simulink model "qpsk"  (Simulink 6.0)
settings: Solver=ode45  StartTime=0.0  StopTime=10.0  RelTol=1e-3
libraries: commsink2 x3, commdigbbndpm2 x2, commchan2 x1, commfilt2 x1, commrandsrc2 x1
settings Model: LastModifiedBy=student

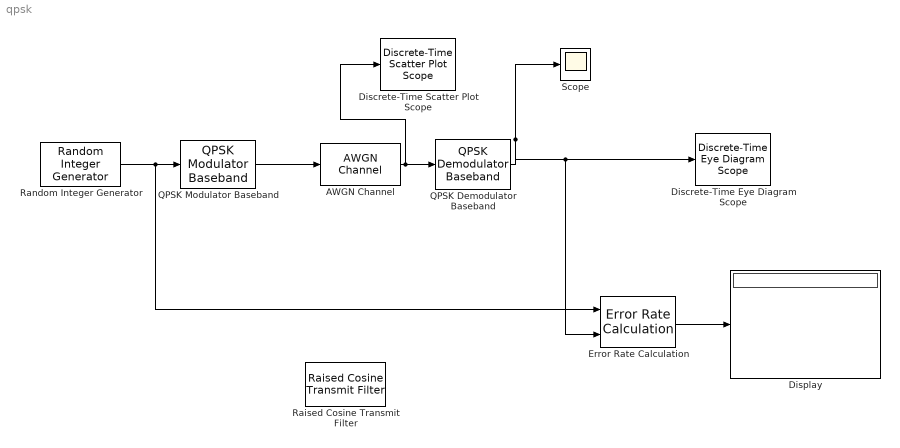
== system qpsk ==
  AWGN Channel : commchan2/AWGN Channel  seed=67  noiseMode="Signal to noise ratio  (Eb/No)"  EbNodB=10  EsNodB=10  SNRdB=10  bitsPerSym=1  Ps=1  Tsym=1  variance=1
  Discrete-Time Eye Diagram Scope : commsink2/Discrete-Time Eye Diagram Scope  Tag=EyeDiagram  sampPerSymb=8  offsetEye=0  symbPerTrace=1  numTraces=40  numNewFrames=10  LineStyles=-  LineColors=b  dupPoints=on  fading=on  render=on  AxisGrid=on  yMin=-1.5  yMax=1.5  inphaseLabel=In-phase Amplitude  quadratureLabel=Quadrature Amplitude  openScopeAtSimStart=on  dispDiagram=In-phase and Quadrature  FrameNumber=off  FigPos=[232 24 560 644]  figTitle=Eye Diagram  block_type_=eye  numLinesMax=8
  Discrete-Time Scatter Plot Scope : commsink2/Discrete-Time Scatter Plot Scope  Tag=ScatterPlot  sampPerSymb=1  offsetEye=0  numTraces=40  numNewFrames=10  LineMarkers=.  LineColors=b  fading=on  render=on  AxisGrid=on  xMin=-1.5  xMax=1.5  yMin=-1.5  yMax=1.5  inphaseLabel=In-phase Amplitude  quadratureLabel=Quadrature Amplitude  openScopeAtSimStart=on  FrameNumber=off  FigPos=[232 108 560 560]  figTitle=Scatter Plot  numLinesMax=8  block_type_=scatter
  Display : Display
  Error Rate Calculation : commsink2/Error Rate Calculation  N=0  st_delay=0  cp_mode=Entire frame  subframe=[]  PMode=Port  WsName=ErrorVec  RsMode2=off  stop=off  numErr=100  maxBits=1e6
  QPSK Demodulator Baseband : commdigbbndpm2/QPSK Demodulator Baseband  OutType=Integer  Dec=Binary  Ph=pi/4  numSamp=1
  QPSK Modulator Baseband : commdigbbndpm2/QPSK Modulator Baseband  InType=Integer  Enc=Binary  Ph=pi/4  numSamp=1
  Raised Cosine Transmit Filter : commfilt2/Raised Cosine Transmit Filter  filtType=Square root  D=4  R=0.2  sampMode=Sample-based  N=8  checkGain=Normalized  filterGain=1  checkCoeff=off  variableName=rcTxFilt  launchFVT=off
  Random Integer Generator : commrandsrc2/Random Integer Generator  mul=4  seed=37  Ts=1  frameBased=off  sampPerFrame=1  orient=off
  Scope : Scope
  wires:
  Random Integer Generator/1 -> QPSK Modulator Baseband/1, Error Rate Calculation/1
  AWGN Channel/1 -> Discrete-Time Scatter Plot Scope/1, QPSK Demodulator Baseband/1
  QPSK Demodulator Baseband/1 -> Scope/1, Discrete-Time Eye Diagram Scope/1, Error Rate Calculation/2
  Error Rate Calculation/1 -> Display/1
  QPSK Modulator Baseband/1 -> AWGN Channel/1
